simulink model "fdcwind"  (Simulink 3.00)
settings: Solver=ode45  StartTime=0.0  StopTime=50.0  RelTol=1e-3
libraries: airlib x1, simulink3 x1
settings Model: ExtModeTrigMode=normal  ExtModeArmWhenConnect=on  LastModifiedBy=gcampa

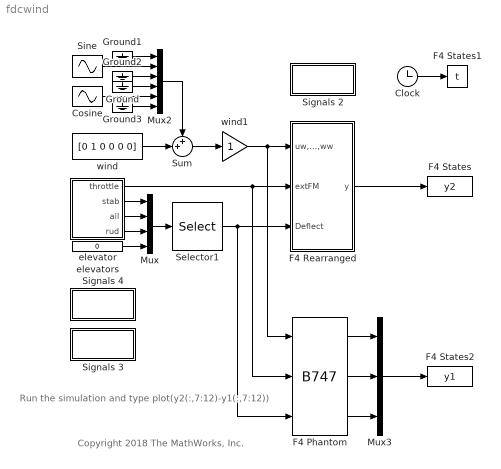
== system fdcwind ==
  note: Run the simulation and type
      | plot(y2(:,7:12)-y1(:,7:12))
  note: Copyright 2018 The MathWorks, Inc.
  " F4 Phantom " : airlib/B747  GM1="[4.8768   11.79576   49.23861   33895.4489   165680.954   189543.35   0   2982.7995  0   17690.1]"  CD_wind="[0.0205  0.3   0  0  -0.1]"  CL_wind="[0.1    3.75    1.8    0    0.4]"  Cm_body="[0.025  -0.4   -2.7    0    -0.58]"  CY_body="[0   -0.68   0     0     0.0160    0.095]"  Cl_body="[0    -0.16    -0.34   0.13    -0.013    0.008]"  Cn_body="[0    0.125   -0.036    -0.270     0.001   -0.066]"  x0="[204.7539671696894 0.0395294 -0.00488392967079  0 0 0   0 0.0395294 0   -70 -20 6065.68]"
  Clock : Clock
      settings: DisplayTime=off  Decimation=10
  Cosine : Sin  Amplitude=1  Frequency=1  Phase=pi/2  SampleTime=0
  F4 Rearranged : Subsystem  mask{GM1=[4.8768   11.79576   49.23861   33895.4489   165680.954   189543.35   0   2982.7995  0   17690.1], CD_wind=[0.0205  0.3   0  0  -0.1], CL_wind=[0.1    3.75    1.8    0    0.4], Cm_body=[0.025  -0.4   -2.7    0    -0.58], CY_body=[0   -0.68   0     0     0.0160    0.095], Cl_body=[0    -0.16    -0.34   0.13    -0.013    0.008], Cn_body=[0    0.125   -0.036    -0.270     0.001   -0.066], x0=[204.7515252  0.0395294 0   0 0 0   0 0.0395294 0   -70 -20 6065.68]}
      mask prompts: GM1 "Geometry and Mass : [cbar   b    S    Ix   Iy   Iz   Jxy  Jxz  Jyz  m]"; CD_wind "Aerodynamic D-Force Coefficients : [CD0 CDa CDq CDde CDih]"; CL_wind "Aerodynamic L-Force Coefficients : [CL0 CLa CLq CLde CLih]"; Cm_body "Aerodynamic Y-Moment Coefficients : [Cm0 Cma Cmq Cmde Cmih]"; CY_body "Aerodynamic Y-Force Coefficients : [CY0 CYb CYp CYr CYda CYdr]"; Cl_body "Aerodynamic X-moment Coefficients : [Cl0 Clb Clp Clr Clda Cldr]"; Cn_body "Aerodynamic Z-moment Coefficients : [Cn0 Cnb Cnp Cnr Cnda Cndr]"; x0 "Initial Condition x0 [v alpha beta p q r psi theta phi xe ye H]"
      mask help:
      | The first input contains the wind velocity and acceleration.
      |   The second input contains external forces and moments in body axis.
      |   The third input contains the deflections of elevators, ailerons, rudder
      |   and, flaps. For a list of outputs look under the mask.
      |   NB : The International measurement system (MKS) is adopted.
      mask init:
      | AM=zeros(6,19);
      | AM(1,[1 2 9 11 12])=reshape(CD_wind,1,5);
      | AM(3,[1 2 9 11 12])=reshape(CL_wind,1,5);
      | AM(5,[1 2 9 11 12])=reshape(Cm_body,1,5);
      | AM(2,[1 5 8 10 13 14])=reshape(CY_body,1,6);
      | AM(4,[1 5 8 10 13 14])=reshape(Cl_body,1,6);
      | AM(6,[1 5 8 10 13 14])=reshape(Cn_body,1,6);
      | 
      | Ix=GM1(4);Iy=GM1(5);Iz=GM1(6);
      | Jxy=GM1(7);Jxz=GM1(8);Jyz=GM1(9);
      | 
      | detI = Ix*Iy*Iz - 2*Jxy*Jxz*Jyz - Ix*Jyz^2 - Iy*Jxz^2 - Iz*Jxy^2;
      | I1   = Iy*Iz - Jyz^2;I2   = Jxy*Iz + Jyz*Jxz;
      | I3   = Jxy*Jyz + Iy*Jxz;I4   = Ix*Iz - Jxz^2;
      | I5   = Ix*Jyz + Jxy*Jxz;I6   = Ix*Iy - Jxy^2;
      | 
      | Pl  = I1/detI; Pm = I2/detI; Pn = I3/detI;
      | Ppp = -(Jxz*I2 - Jxy*I3)/detI;Ppq = (Jxz*I1 - Jyz*I2 - (Iy-Ix)*I3)/detI;
      | Ppr = -(Jxy*I1 + (Ix-Iz)*I2 - Jyz*I3)/detI;Pqq = (Jyz*I1 - Jxy*I3)/detI;
      | Pqr = -((Iz-Iy)*I1 - Jxy*I2 + Jxz*I3)/detI;Prr = -(Jyz*I1 - Jxz*I2)/detI;
      | 
      | Ql  = I2/detI; Qm = I4/detI; Qn = I5/detI;
      | Qpp = -(Jxz*I4 - Jxy*I5)/detI;Qpq = (Jxz*I2 - Jyz*I4 - (Iy-Ix)*I5)/detI;
      | Qpr = -(Jxy*I2 + (Ix-Iz)*I4 - Jyz*I5)/detI;Qqq = (Jyz*I2 - Jxy*I5)/detI;
      | Qqr = -((Iz-Iy)*I2 - Jxy*I4 + Jxz*I5)/detI;Qrr = -(Jyz*I2 - Jxz*I4)/detI;
      | 
      | Rl  = I3/detI; Rm = I5/detI; Rn = I6/detI;
      | Rpp = -(Jxz*I5 - Jxy*I6)/detI;
      | Rpq = (Jxz*I3 - Jyz*I5 - (Iy-Ix)*I6)/detI;
      | Rpr = -(Jxy*I3 + (Ix-Iz)*I5 - Jyz*I6)/detI;
      | Rqq = (Jyz*I3 - Jxy*I6)/detI;
      | Rqr = -((Iz-Iy)*I3 - Jxy*I5 + Jxz*I6)/detI;
      | Rrr = -(Jyz*I3 - Jxz*I5)/detI;
      | 
      | GM2 = [  Pl   Pm   Pn   Ppp  Ppq  Ppr  Pqq  Pqr  Prr ;
      |                Ql  Qm   Qn   Qpp  Qpq  Qpr  Qqq  Qqr  Qrr ;
      |                Rl  Rm   Rn   Rpp  Rpq  Rpr  Rqq  Rqr  Rrr ];
      | 
      | xfix=1;
  F4 States : ToWorkspace  VariableName=y2  SampleTime=0.05  SaveFormat=Matrix
      settings: Buffer=1000
  F4 States1 : ToWorkspace  VariableName=t  SampleTime=0.05  SaveFormat=Matrix
      settings: Buffer=1000
  F4 States2 : ToWorkspace  VariableName=y1  SampleTime=0.05  SaveFormat=Matrix
      settings: Buffer=1000
  Ground{,1..3} (4 alike) : Ground
  Mux : Mux  Inputs=4
      settings: DisplayOption=none
  Mux2 : Mux  Inputs=[1,1,1,1,1,1]
      settings: DisplayOption=none
  Mux3 : Mux  Inputs=3
      settings: DisplayOption=none
  Selector1 : Selector  Elements=[4 2 3 1]  InputPortWidth=4
  Signals 2 : Subsystem
      mask Display: disp('Model \nSignals')
  Signals 3 : Subsystem
      mask Display: disp('Initial \nConditions')
  Signals 4 : Subsystem
      mask Display: disp('INFO')
  Sine : Sin  Amplitude=1  Frequency=1  Phase=0  SampleTime=0
  Sum : Sum  Inputs=++|  SaturateOnIntegerOverflow=on
  elevator : Subsystem
      mask Display: disp('Cable &\nactuator\ndynamics')
  elevators : Constant  Value=0
  wind : Constant  Value=[0 1 0 0 0 0]
  wind1 : Gain  Gain=1  SaturateOnIntegerOverflow=on
  wires:
  elevator/3(ail) -> Mux/2
  elevator/4(rud) -> Mux/3
  elevator/2(stab) -> Mux/1
  Mux/1 -> Selector1/1
  elevators/1 -> Mux/4
  elevator/1(throttle) -> F4 Rearranged/2(extFM), " F4 Phantom "/2
  Selector1/1 -> F4 Rearranged/3(Deflect), " F4 Phantom "/3
  Mux3/1 -> F4 States2/1
  F4 Rearranged/1(y) -> F4 States/1
  wind/1 -> Sum/2
  Clock/1 -> F4 States1/1
  Sine/1 -> Mux2/2
  Ground1/1 -> Mux2/1
  Ground2/1 -> Mux2/3
  Ground/1 -> Mux2/4
  Ground3/1 -> Mux2/6
  Cosine/1 -> Mux2/5
  Mux2/1 -> Sum/1
  Sum/1 -> wind1/1
  wind1/1 -> F4 Rearranged/1(uw,vw,ww), " F4 Phantom "/1
  " F4 Phantom "/1 -> Mux3/1
  " F4 Phantom "/2 -> Mux3/2
  " F4 Phantom "/3 -> Mux3/3

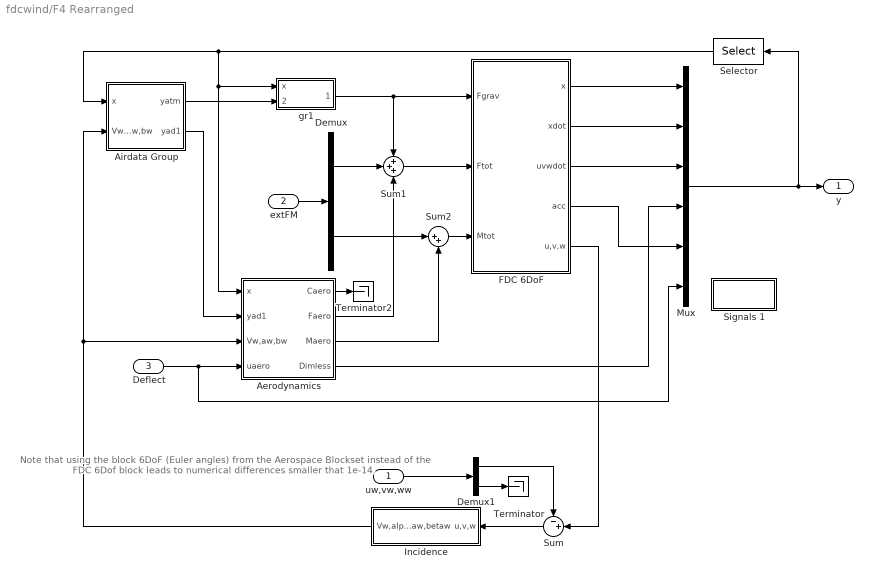
== system fdcwind/F4 Rearranged ==
  note: Note that using the block 6DoF (Euler angles)
      | from the Aerospace Blockset instead of the
      | FDC 6Dof block leads to numerical differences
      | smaller that 1e-14.
  uw,vw,ww : Inport  Port=1  PortWidth=6  SampleTime=-1  DataType=auto
      settings: SignalType=auto
  extFM : Inport  Port=2  PortWidth=6  SampleTime=-1  DataType=auto
      settings: SignalType=auto
  Deflect : Inport  Port=3  PortWidth=-1  SampleTime=-1  DataType=auto
      settings: SignalType=auto
  Aerodynamics : Subsystem
  Airdata Group : Subsystem
  Demux : Demux  Outputs=[3,3]
  Demux1 : Demux  Outputs=[3,3]
  FDC 6DoF : Subsystem
  Incidence : Subsystem  Orientation=left
  Mux : Mux  Inputs=6
  Selector : Selector  Orientation=left  Elements=[1:12]  InputPortWidth=40
  Signals 1 : Subsystem
      mask Display: disp('Output\nSignals')
  Sum : Sum  Orientation=left  Inputs=-+|  SaturateOnIntegerOverflow=on
  Sum1 : Sum  Inputs=+++  SaturateOnIntegerOverflow=on
  Sum2 : Sum  Inputs=|++  SaturateOnIntegerOverflow=on
  Terminator : Terminator
  Terminator2 : Terminator
  gr1 : Subsystem  mask(Gravity){m=GM1(10)}
      mask prompts: m "Mass of the aircraft [kg]:"
      mask help: Gravity forces.
      mask Help: eval('fdchelp gravity')
      mask Display: disp('Gravity')
  y : Outport  Port=1
  wires:
  Aerodynamics/4(Dimless) -> Mux/4
  FDC 6DoF/4(acc) -> Mux/5
  FDC 6DoF/3(uvwdot) -> Mux/3
  FDC 6DoF/2(xdot) -> Mux/2
  FDC 6DoF/1(x) -> Mux/1
  Sum1/1 -> FDC 6DoF/2(Ftot)
  Demux1/2 -> Terminator/1
  Demux1/1 -> Sum/1
  uw,vw,ww/1 -> Demux1/1
  Selector/1 -> Airdata Group/1(x), gr1/1(x), Aerodynamics/1(x)
  Mux/1 -> Selector/1, y/1
  Sum2/1 -> FDC 6DoF/3(Mtot)
  Demux/2 -> Sum2/1
  Aerodynamics/1(Caero) -> Terminator2/1
  Deflect/1 -> Mux/6, Aerodynamics/4(uaero)
  Airdata Group/2(yad1) -> Aerodynamics/2(yad1)
  Incidence/1(Vw,alphaw,betaw) -> Aerodynamics/3(Vw,aw,bw), Airdata Group/2(Vw,aw,bw)
  Sum/1 -> Incidence/1(u,v,w)
  Airdata Group/1(yatm) -> gr1/2(yatm)
  gr1/1(Fgrav) -> FDC 6DoF/1(Fgrav), Sum1/1
  FDC 6DoF/5(u,v,w) -> Sum/2
  extFM/1 -> Demux/1
  Demux/1 -> Sum1/2
  Aerodynamics/2(Faero) -> Sum1/3
  Aerodynamics/3(Maero) -> Sum2/2

== system fdcwind/Signals 2 ==
  note: 01 v (m/s)
      | 02 alpha (rad)
      | 03 beta (rad)
      | 04 p (rad/s)
      | 05 q (rad/s)
      | 06 r  (rad/s)
      | 07 psi (rad)
      | 08 theta (rad)
      | 09 phi (rad)
      | 10 xe (m)
      | 11 ye (m)
      | 12 H (m)
      | 13 v dot (m/s2)
      | 14 alpha dot (rad/s)
      | 15 beta dot (rad/s)
      | 16 p dot (rad/s2)
      | 17 q dot (rad/s2)
      | 18 r dot (rad/s2)
      | 19 psi dot (rad/s)
      | 20 theta dot (rad/s)
      | 21 phi dot (rad/s)
      | 22 xe dot (m/s)
      | 23 ye dot (m/s)
      | 24 H dot (m/s)
      | 25 u dot (m/s2)
      | 26 v dot (m/s2)
      | 27 w dot (m/s2)
      | 28 pb/2v (rad)
      | 29 qc/v (rad)
      | 30 rb/v (rad)
      | 31 Ax (g)
      | 32 Ay (g)
      | 33 Az (g)
      | 34 ax (g)
      | 35 ay (g)
      | 36 az (g)
      | 37 delta elevators (rad)
      | 38 delta ailerons (rad)
      | 39 delta rudder (rad)
      | 40 delta flaps (rad)

== system fdcwind/Signals 3 ==
  note: V=204.7515252;a=0.0395294;b=0;
      | u=V*cos(a)*cos(b);v=V*sin(b);w=V*sin(a)*cos(b);
      |
      | uw=0;vw=1;ww=0;
      |
      | Vw=norm([u v w]-[uw vw ww]);
      | aw=atan((w-ww)/(u-uw));
      | bw=atan((v-vw)/norm([u w]-[uw ww]));
  note: INITIAL CONDITION COMPUTATION FOR
      | THE FDC AIRCRAFT MODEL WITH NONZERO
      | INITIAL WIND

== system fdcwind/Signals 4 ==
  note: This scheme compares two different but
      | equivalent ways to handle the wind
      | inside the equations of motions.
      |
      |
      | It also proves that the way in which FDC handles
      | the wind is fully correct provided that the right
      | initial conditions are chosen for V,alpha,beta
      | whenever the initial value of the wind is nonzero.

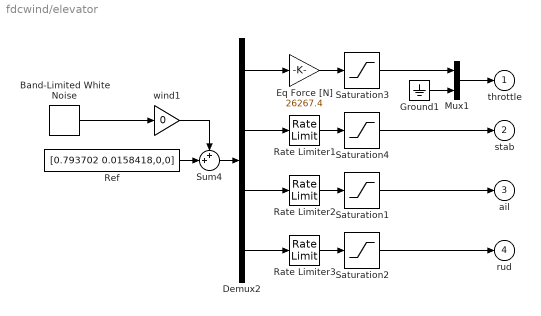
== system fdcwind/elevator ==
  Band-Limited White Noise : simulink3/Sources/Band-Limited White Noise  Cov=0.1*ones(1,4)  Ts=0.1  seed=[1 2 3 4]
  Demux2 : Demux  Outputs=4
  Eq Force [N] : Gain  Gain=26267.4  SaturateOnIntegerOverflow=on
  Ground1 : Ground
  Mux1 : Mux  Inputs=[1 5]
      settings: DisplayOption=none
  Rate Limiter1 : RateLimiter  RisingSlewLimit=100*pi/180  FallingSlewLimit=-100*pi/180
  Rate Limiter2 : RateLimiter  RisingSlewLimit=100*pi/180  FallingSlewLimit=-100*pi/180
  Rate Limiter3 : RateLimiter  RisingSlewLimit=100*pi/180  FallingSlewLimit=-100*pi/180
  Ref : Constant  Value=[0.793702 0.0158418,0,0]
  Saturation1 : Saturate  UpperLimit=20*pi/180  LowerLimit=-20*pi/180
  Saturation2 : Saturate  UpperLimit=20*pi/180  LowerLimit=-20*pi/180
  Saturation3 : Saturate  UpperLimit=52534.8  LowerLimit=0
  Saturation4 : Saturate  UpperLimit=20*pi/180  LowerLimit=-20*pi/180
  Sum4 : Sum  Inputs=++|  SaturateOnIntegerOverflow=on
  wind1 : Gain  Gain=0  SaturateOnIntegerOverflow=on
  throttle : Outport  Port=1
  stab : Outport  Port=2
  ail : Outport  Port=3
  rud : Outport  Port=4
  wires:
  Eq Force [N]/1 -> Saturation3/1
  Ground1/1 -> Mux1/2
  Mux1/1 -> throttle/1
  Saturation3/1 -> Mux1/1
  Ref/1 -> Sum4/2
  Sum4/1 -> Demux2/1
  Rate Limiter1/1 -> Saturation4/1
  Saturation4/1 -> stab/1
  Rate Limiter2/1 -> Saturation1/1
  Saturation1/1 -> ail/1
  Rate Limiter3/1 -> Saturation2/1
  Saturation2/1 -> rud/1
  Demux2/4 -> Rate Limiter3/1
  Demux2/3 -> Rate Limiter2/1
  Demux2/2 -> Rate Limiter1/1
  Demux2/1 -> Eq Force [N]/1
  Band-Limited White Noise/1 -> wind1/1
  wind1/1 -> Sum4/1

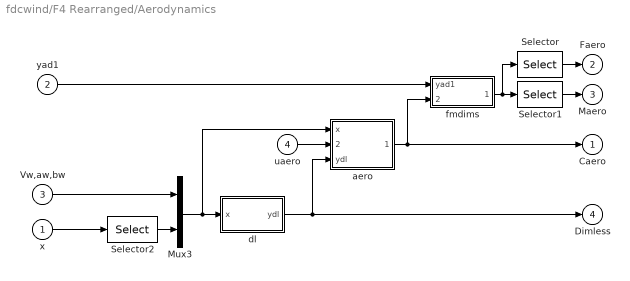
== system fdcwind/F4 Rearranged/Aerodynamics ==
  x : Inport  Port=1  PortWidth=-1  SampleTime=-1  DataType=auto
      settings: SignalType=auto
  yad1 : Inport  Port=2  PortWidth=-1  SampleTime=-1  DataType=auto
      settings: SignalType=auto
  Vw,aw,bw : Inport  Port=3  PortWidth=3  SampleTime=-1  DataType=auto
      settings: SignalType=auto
  uaero : Inport  Port=4  PortWidth=-1  SampleTime=-1  DataType=auto
      settings: SignalType=auto
  Mux3 : Mux  Inputs=2
  Selector : Selector  Elements=[1:3]  InputPortWidth=6
  Selector1 : Selector  Elements=[4:6]  InputPortWidth=6
  Selector2 : Selector  Elements=[4:12]  InputPortWidth=12
  aero : Subsystem
      mask Type: Aeromod
      mask Description: Aerodynamic model of the DHC-2 'Beaver'.
      mask Help: eval('fdchelp aeromod')
      mask Display: disp('Aeromod\n(General)')
  dl : Subsystem  mask(Dimless){cbar=GM1(1), b=GM1(2)}
      mask prompts: cbar "Mean aerodynamic chord [m]:"; b "Wing span [m]:"
      mask help: Dimensionless rotational velocities.
      mask Help: eval('fdchelp dimless')
      mask Display: disp('Dimless')
  fmdims : Subsystem  mask(FMdims){cbar=GM1(1), b=GM1(2), S=GM1(3)}
      mask prompts: cbar "Mean aerodynamic chord [m]:"; b "Wing span [m]:"; S "Wing surface [m^2]:"
      mask help:
      | Calculate forces and moments from
      | dimensionless coefficients.
      mask Help: eval('fdchelp fmdims')
      mask Display: disp('FMdims')
  Caero : Outport  Port=1
  Faero : Outport  Port=2
  Maero : Outport  Port=3
  Dimless : Outport  Port=4
  wires:
  Selector2/1 -> Mux3/2
  Vw,aw,bw/1 -> Mux3/1
  x/1 -> Selector2/1
  Mux3/1 -> aero/1(x), dl/1(x)
  dl/1(ydl) -> Dimless/1, aero/3(ydl)
  aero/1(Caero) -> fmdims/2(Force / moment coefficients), Caero/1
  uaero/1 -> aero/2(uaero)
  yad1/1 -> fmdims/1(yad1)
  fmdims/1(Forces and moments) -> Selector1/1, Selector/1
  Selector1/1 -> Maero/1
  Selector/1 -> Faero/1

== system fdcwind/F4 Rearranged/Airdata Group ==
  x : Inport  Port=1  PortWidth=12  SampleTime=-1  DataType=auto
      settings: SignalType=auto
  Vw,aw,bw : Inport  Port=2  PortWidth=3  SampleTime=-1  DataType=auto
      settings: SignalType=auto
  ad1 : Subsystem
      mask Type: Airdata1
      mask Description: Basic airdata variables
      mask Help: eval('fdchelp airdata1')
      mask Display: disp('Airdata1')
  atm1 : Subsystem
      mask Type: Atmosph
      mask Description:
      | 1-Atmosphere variables
      | 2-Air density
      | 3-Air Pressure
      | 4-Temperature
      | 5-Air viscosity
      | 6-Gravity
      mask Help: eval('fdchelp atmosph')
      mask Display: disp('Atmosph')
  yatm : Outport  Port=1
  yad1 : Outport  Port=2
  wires:
  Vw,aw,bw/1 -> ad1/1(Vw,alphaw,betaw)
  ad1/1(yad1) -> yad1/1
  atm1/1(yatm) -> yatm/1, ad1/2(yatm)
  x/1 -> atm1/1(x)

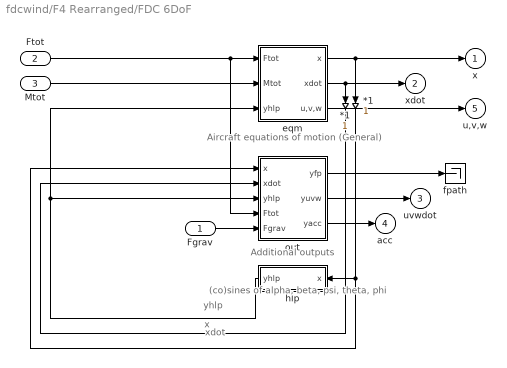
== system fdcwind/F4 Rearranged/FDC 6DoF ==
  note: (co)sines of
      | alpha, beta,
      | psi, theta, phi
  note: Aircraft equations
      | of motion (General)
  note: Additional outputs
  note: yhlp
  note: x
  note: xdot
  Fgrav : Inport  Port=1  PortWidth=3  SampleTime=-1  DataType=auto
      settings: SignalType=auto
  Ftot : Inport  Port=2  PortWidth=3  SampleTime=-1  DataType=auto
      settings: SignalType=auto
  Mtot : Inport  Port=3  PortWidth=3  SampleTime=-1  DataType=auto
      settings: SignalType=auto
  " *1" : Gain  Orientation=down  Gain=1  SaturateOnIntegerOverflow=on
  *1 : Gain  Orientation=down  Gain=1  SaturateOnIntegerOverflow=on
  eqm : Subsystem
  fpath : Terminator
  hlp : Subsystem  Orientation=left
      mask Type: Hlpfcn
      mask Description: Help sines and cosines
      mask Help: eval('fdchelp hlpfcn')
      mask Display: disp('hlpfcn')
  out : Subsystem
  x : Outport  Port=1
  xdot : Outport  Port=2
  uvwdot : Outport  Port=3
  acc : Outport  Port=4
  u,v,w : Outport  Port=5
  wires:
  eqm/3(u,v,w) -> u,v,w/1
  Fgrav/1 -> out/5(Fgrav)
  eqm/2(xdot) -> *1/1, xdot/1
  Mtot/1 -> eqm/2(Mtot)
  Ftot/1 -> eqm/1(Ftot), out/4(Ftot)
  eqm/1(x) -> " *1"/1, x/1
  " *1"/1 -> out/1(x), hlp/1(x)
  out/3(yacc) -> acc/1
  out/1(yfp) -> fpath/1
  out/2(yuvw) -> uvwdot/1
  *1/1 -> out/2(xdot)
  hlp/1(yhlp) -> out/3(yhlp), eqm/3(yhlp)

== system fdcwind/F4 Rearranged/Incidence ==
  u,v,w : Inport  Port=1  PortWidth=3  SampleTime=-1  DataType=auto
      settings: SignalType=auto
  Mux2 : Mux  Inputs=3
  Vrel : Fcn  Expr=sqrt(u[1]^2+u[2]^2+u[3]^2)
  alpha app : Fcn  Expr=atan2(u[3],u[1])
  beta app : Fcn  Expr=atan2(u[2],sqrt(u[1]^2+u[3]^2))
  Vw,alphaw,betaw : Outport  Port=1
  wires:
  Mux2/1 -> Vw,alphaw,betaw/1
  u,v,w/1 -> Vrel/1, alpha app/1, beta app/1
  beta app/1 -> Mux2/3
  alpha app/1 -> Mux2/2
  Vrel/1 -> Mux2/1

== system fdcwind/F4 Rearranged/Signals 1 ==
  note: 01 v (m/s)                        1
      | 02 alpha (rad)                 2
      | 03 beta (rad)                   3
      | 04 p (rad/s)                      4
      | 05 q (rad/s)                      5
      | 06 r  (rad/s)                      6
      | 07 psi (rad)                      7
      | 08 theta (rad)                  8
      | 09 phi (rad)                     9
      | 10 xe (m)
      | 11 ye (m)
      | 12 ze (m)
      | 13 v dot (m/s2)
      | 14 alpha dot (rad/s)
      | 15 beta dot (rad/s)
      | 16 p dot (rad/s2)
      | 17 q dot (rad/s2)
      | 18 r dot (rad/s2)
      | 19 fi dot (rad/s)
      | 20 theta dot (rad/s)
      | 21 psi dot (rad/s)
      | 22 xe dot (m/s)
      | 23 ye dot (m/s)
      | 24 ze dot (m/s)
      | 25 u dot (m/s2)               10
      | 26 v dot (m/s2)               11
      | 27 w dot (m/s2)              12
      | 28 pb/2v (rad)
      | 29 qc/v (rad)
      | 30 rb/v (rad)
      | 31 Ax (g)                        13
      | 32 Ay (g)                        14
      | 33 Az (g)                        15
      | 34 ax (g)                        16
      | 35 ay (g)                        17
      | 36 az (g)                        18
      | 37 delta elevators (rad)  19
      | 38 delta ailerons (rad)    20
      | 39 delta rudder (rad)      21
      | 40 delta flaps (rad)

== system fdcwind/F4 Rearranged/gr1 ==
  x : Inport  Port=1  PortWidth=-1  SampleTime=-1  DataType=auto
      settings: SignalType=auto
  yatm : Inport  Port=2  PortWidth=-1  SampleTime=-1  DataType=auto
      settings: SignalType=auto
  0 : Subsystem
      settings: OpenFcn=fdchelp gravity
      mask Display: disp('GRAVITY\nM.O. Rauw, October 1997')
  Mux : Mux  Inputs=3
      settings: DisplayOption=none
  Mux1 : Mux  Inputs=[12 5]
      settings: DisplayOption=none
  Xgr : Fcn  Expr=-m*u[17]*sin(u[8])
  Ygr : Fcn  Expr=m*u[17]*cos(u[8])*sin(u[9])
  Zgr : Fcn  Expr=m*u[17]*cos(u[8])*cos(u[9])
  Fgrav : Outport  Port=1
  wires:
  yatm/1 -> Mux1/2
  x/1 -> Mux1/1
  Zgr/1 -> Mux/3
  Mux1/1 -> Zgr/1, Xgr/1, Ygr/1
  Mux/1 -> Fgrav/1
  Ygr/1 -> Mux/2
  Xgr/1 -> Mux/1

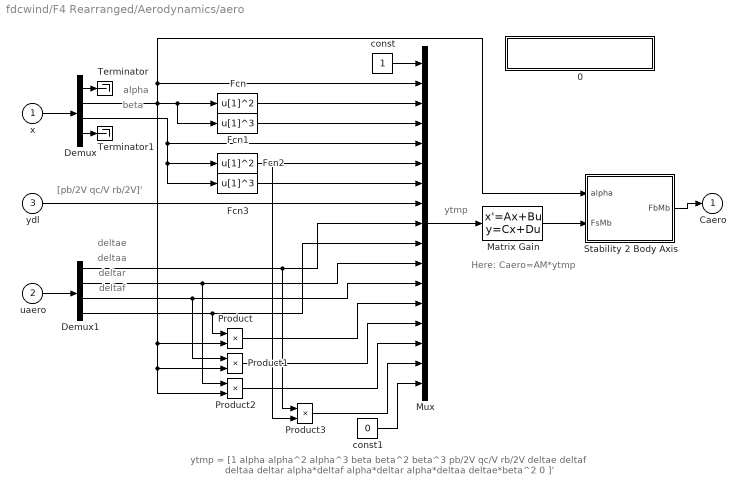
== system fdcwind/F4 Rearranged/Aerodynamics/aero ==
  note: Here: Caero=AM*ytmp
  note: ytmp
  note: alpha
  note: deltaf
  note: deltar
  note: deltaa
  note: deltae
  note: beta
  note: [pb/2V qc/V rb/2V]'
  note: ytmp = [1  alpha  alpha^2  alpha^3  beta  beta^2  beta^3  pb/2V  qc/V  rb/2V  deltae
      | deltaf  deltaa  deltar  alpha*deltaf  alpha*deltar  alpha*deltaa  deltae*beta^2  0 ]'
  x : Inport  Port=1  PortWidth=-1  SampleTime=-1  DataType=auto
      settings: SignalType=auto
  uaero : Inport  Port=2  PortWidth=-1  SampleTime=-1  DataType=auto
      settings: SignalType=auto
  ydl : Inport  Port=3  PortWidth=-1  SampleTime=-1  DataType=auto
      settings: SignalType=auto
  0 : Subsystem
      settings: OpenFcn=fdchelp aeromod
      mask Display: disp('AEROMOD\nM.O. Rauw, October 1997')
  Demux : Demux  Outputs=[1 1 1 9]
  Demux1 : Demux  Outputs=4
  Fcn : Fcn  Expr=u[1]^2
  Fcn1 : Fcn  Expr=u[1]^3
  Fcn2 : Fcn  Expr=u[1]^2
  Fcn3 : Fcn  Expr=u[1]^3
  Matrix Gain : StateSpace  A=[]  B=[]  C=[]  D=AM  X0=0
  Mux : Mux  Inputs=[1 1 1 1 1 1 1 3 1 1 1 1 1 1 1 1 1]
      settings: DisplayOption=none
  Product{,1..3} (4 alike) : Product  Inputs=2  SaturateOnIntegerOverflow=on
  Stability 2 Body Axis : Subsystem
  Terminator : Terminator
  Terminator1 : Terminator
  const : Constant  Value=1
  const1 : Constant  Value=0
  Caero : Outport  Port=1
  wires:
  Matrix Gain/1 -> Stability 2 Body Axis/2(FsMb)
  Stability 2 Body Axis/1(FbMb) -> Caero/1
  Mux/1 -> Matrix Gain/1
  x/1 -> Demux/1
  Fcn/1 -> Mux/3
  Fcn1/1 -> Mux/4
  uaero/1 -> Demux1/1
  Fcn3/1 -> Mux/7
  Product/1 -> Mux/13
  Demux1/3 -> Product1/1, Mux/12
  Demux1/2 -> Product2/1, Mux/11
  Demux/3 -> Fcn3/1, Fcn2/1, Mux/5
  Demux/2 -> Stability 2 Body Axis/1(alpha), Mux/2, Product2/2, Product1/2, Product/2, Fcn1/1, Fcn/1
  Demux1/4 -> Product/1, Mux/10
  Fcn2/1 -> Product3/2, Mux/6
  Demux1/1 -> Product3/1, Mux/9
  Product1/1 -> Mux/14
  Product2/1 -> Mux/15
  Product3/1 -> Mux/16
  ydl/1 -> Mux/8
  const/1 -> Mux/1
  const1/1 -> Mux/17
  Demux/1 -> Terminator/1
  Demux/4 -> Terminator1/1

== system fdcwind/F4 Rearranged/Aerodynamics/dl ==
  x : Inport  Port=1  PortWidth=-1  SampleTime=-1  DataType=auto
      settings: SignalType=auto
  0 : Subsystem
      settings: OpenFcn=fdchelp dimless
      mask Display: disp('DIMLESS\nM.O. Rauw, October 1997')
  Mux : Mux  Inputs=3
      settings: DisplayOption=none
  pb/2V : Fcn  Expr=0.5 * u[4] * b / u[1]
  qc/2V : Fcn  Expr=0.5* u[5] * cbar / u[1]
  rb/2V : Fcn  Expr=0.5 * u[6] * b / u[1]
  ydl : Outport  Port=1
  wires:
  x/1 -> pb/2V/1, rb/2V/1, qc/2V/1
  Mux/1 -> ydl/1
  rb/2V/1 -> Mux/3
  qc/2V/1 -> Mux/2
  pb/2V/1 -> Mux/1

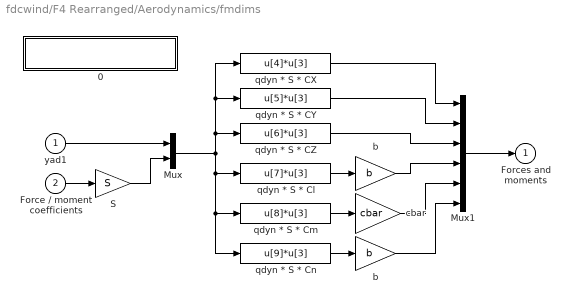
== system fdcwind/F4 Rearranged/Aerodynamics/fmdims ==
  yad1 : Inport  Port=1  PortWidth=-1  SampleTime=-1  DataType=auto
      settings: SignalType=auto
  Force / moment coefficients : Inport  Port=2  PortWidth=-1  SampleTime=-1  DataType=auto
      settings: SignalType=auto
  0 : Subsystem
      settings: OpenFcn=fdchelp fmdims
      mask Display: disp('FMDIMS\nM.O. Rauw, October 1997')
  Mux : Mux  Inputs=[3 6]
      settings: DisplayOption=none
  Mux1 : Mux  Inputs=6
      settings: DisplayOption=none
  S : Gain  Gain=S  SaturateOnIntegerOverflow=on
  b : Gain  Gain=b  SaturateOnIntegerOverflow=on
  "b " : Gain  Gain=b  SaturateOnIntegerOverflow=on
  cbar : Gain  Gain=cbar  SaturateOnIntegerOverflow=on
  qdyn * S * CX : Fcn  Expr=u[4]*u[3]
  qdyn * S * CY : Fcn  Expr=u[5]*u[3]
  qdyn * S * CZ : Fcn  Expr=u[6]*u[3]
  qdyn * S * Cl : Fcn  Expr=u[7]*u[3]
  qdyn * S * Cm : Fcn  Expr=u[8]*u[3]
  qdyn * S * Cn : Fcn  Expr=u[9]*u[3]
  Forces and moments : Outport  Port=1
  wires:
  b/1 -> Mux1/4
  qdyn * S * CZ/1 -> Mux1/3
  S/1 -> Mux/2
  qdyn * S * CY/1 -> Mux1/2
  qdyn * S * CX/1 -> Mux1/1
  yad1/1 -> Mux/1
  qdyn * S * Cn/1 -> "b "/1
  qdyn * S * Cm/1 -> cbar/1
  qdyn * S * Cl/1 -> b/1
  Mux/1 -> qdyn * S * Cn/1, qdyn * S * Cm/1, qdyn * S * Cl/1, qdyn * S * CY/1, qdyn * S * CX/1, qdyn * S * CZ/1
  Force / moment coefficients/1 -> S/1
  cbar/1 -> Mux1/5
  "b "/1 -> Mux1/6
  Mux1/1 -> Forces and moments/1

== system fdcwind/F4 Rearranged/Airdata Group/ad1 ==
  Vw,alphaw,betaw : Inport  Port=1  PortWidth=-1  SampleTime=-1  DataType=auto
      settings: SignalType=auto
  yatm : Inport  Port=2  PortWidth=-1  SampleTime=-1  DataType=auto
      settings: SignalType=auto
  0 : Subsystem
      settings: OpenFcn=fdchelp airdata1
      mask Display: disp('AIRDATA1\nM.O. Rauw, October 1997')
  M : Fcn  Expr=u[2]/u[1]
  Mux : Mux  Inputs=[1 3]
      settings: DisplayOption=none
  Mux1 : Mux  Inputs=[3 5]
      settings: DisplayOption=none
  Mux2 : Mux  Inputs=3
      settings: DisplayOption=none
  a : Fcn  Expr=sqrt(401.8743*u[3])
  qdyn : Fcn  Expr=0.5*u[4]*u[1]^2
  yad1 : Outport  Port=1
  wires:
  yatm/1 -> Mux1/2, a/1
  Vw,alphaw,betaw/1 -> Mux1/1, Mux/2
  Mux/1 -> M/1
  Mux1/1 -> qdyn/1
  M/1 -> Mux2/2
  a/1 -> Mux2/1, Mux/1
  qdyn/1 -> Mux2/3
  Mux2/1 -> yad1/1

== system fdcwind/F4 Rearranged/Airdata Group/atm1 ==
  x : Inport  Port=1  PortWidth=-1  SampleTime=-1  DataType=auto
      settings: SignalType=auto
  0 : Subsystem
      settings: OpenFcn=fdchelp atmosph
      mask Display: disp('ATMOSPH\nM.O. Rauw, October 1997')
  Mux : Mux  Inputs=2
      settings: DisplayOption=none
  Mux1 : Mux  Inputs=[2 1]
      settings: DisplayOption=none
  Mux2 : Mux  Inputs=5
      settings: DisplayOption=none
  T : Fcn  Expr=288.15 - 0.0065*u[12]
  g : Fcn  Expr=9.80665*(6371020/(6371020+u[12]))^2
  mu : Fcn  Expr=(1.458*10^(-6)*u[2]^1.5)/(u[2]+110.4)
  ps : Fcn  Expr=101325*(u[2]/288.15)^(u[1]/1.86584)
  rho : Fcn  Expr=u[3]/(287.053*u[2])
  yatm : Outport  Port=1
  wires:
  mu/1 -> Mux2/4
  Mux2/1 -> yatm/1
  Mux1/1 -> rho/1
  rho/1 -> Mux2/1
  g/1 -> Mux2/5, Mux/1
  T/1 -> Mux2/3, Mux/2
  ps/1 -> Mux2/2, Mux1/2
  Mux/1 -> ps/1, mu/1, Mux1/1
  x/1 -> g/1, T/1

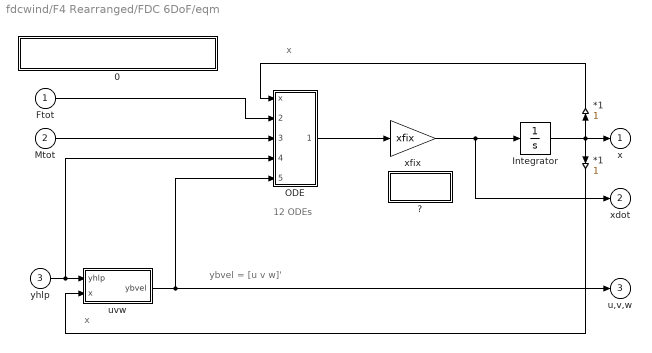
== system fdcwind/F4 Rearranged/FDC 6DoF/eqm ==
  note: 12 ODEs
  note: ybvel = [u v w]'
  note: x
  note: x
  Ftot : Inport  Port=1  PortWidth=-1  SampleTime=-1  DataType=auto
      settings: SignalType=auto
  Mtot : Inport  Port=2  PortWidth=-1  SampleTime=-1  DataType=auto
      settings: SignalType=auto
  yhlp : Inport  Port=3  PortWidth=-1  SampleTime=-1  DataType=auto
      settings: SignalType=auto
  " *1" : Gain  Orientation=up  Gain=1  SaturateOnIntegerOverflow=on
  *1 : Gain  Orientation=down  Gain=1  SaturateOnIntegerOverflow=on
  0 : Subsystem
      settings: OpenFcn=fdchelp eqmotion
      mask Display: disp('EQUATIONS OF MOTION (level 3)\nM.O. Rauw')
  "?" : Subsystem
      settings: OpenFcn=fdchelp xfix
      mask Display: disp('More info\nfor xfix')
  Integrator : Integrator  ExternalReset=none  InitialConditionSource=internal  InitialCondition=x0  LimitOutput=off  UpperSaturationLimit=inf  LowerSaturationLimit=-inf  ShowSaturationPort=off  ShowStatePort=off  AbsoluteTolerance=auto
  ODE : Subsystem
  uvw : Subsystem
      mask Type: uvw
      mask Description:
      | Calculation of body-axes velocities
      | u, v, and w
      mask Help: eval('fdchelp uvw')
      mask Display: disp('Body-axes\nvelocities')
  xfix : Gain  Gain=xfix  SaturateOnIntegerOverflow=on
  x : Outport  Port=1
  xdot : Outport  Port=2
  u,v,w : Outport  Port=3
  wires:
  *1/1 -> uvw/2(x)
  Mtot/1 -> ODE/3(Mtot)
  Ftot/1 -> ODE/2(Ftot)
  uvw/1(ybvel) -> ODE/5(ybvel*), u,v,w/1
  yhlp/1 -> uvw/1(yhlp), ODE/4(yhlp)
  " *1"/1 -> ODE/1(x)
  Integrator/1 -> *1/1, " *1"/1, x/1
  ODE/1(xdot) -> xfix/1
  xfix/1 -> Integrator/1, xdot/1

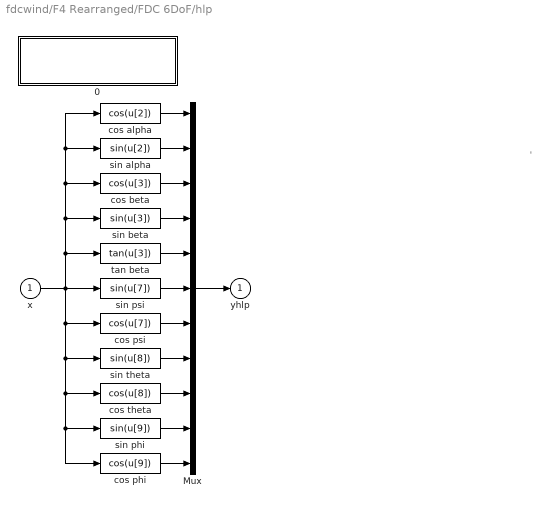
== system fdcwind/F4 Rearranged/FDC 6DoF/hlp ==
  note: '
  x : Inport  Port=1  PortWidth=-1  SampleTime=-1  DataType=auto
      settings: SignalType=auto
  0 : Subsystem
      settings: OpenFcn=fdchelp hlpfcn
      mask Display: disp('HELP FUNCTIONS\n(often used sines and cosines)\nM.O. Rauw, October 1997')
  Mux : Mux  Inputs=11
      settings: DisplayOption=none
  cos alpha : Fcn  Expr=cos(u[2])
  cos beta : Fcn  Expr=cos(u[3])
  cos phi : Fcn  Expr=cos(u[9])
  cos psi : Fcn  Expr=cos(u[7])
  cos theta : Fcn  Expr=cos(u[8])
  sin alpha : Fcn  Expr=sin(u[2])
  sin beta : Fcn  Expr=sin(u[3])
  sin phi : Fcn  Expr=sin(u[9])
  sin psi : Fcn  Expr=sin(u[7])
  sin theta : Fcn  Expr=sin(u[8])
  tan beta : Fcn  Expr=tan(u[3])
  yhlp : Outport  Port=1
  wires:
  cos phi/1 -> Mux/11
  Mux/1 -> yhlp/1
  sin phi/1 -> Mux/10
  cos theta/1 -> Mux/9
  sin theta/1 -> Mux/8
  cos psi/1 -> Mux/7
  sin psi/1 -> Mux/6
  tan beta/1 -> Mux/5
  sin beta/1 -> Mux/4
  cos beta/1 -> Mux/3
  sin alpha/1 -> Mux/2
  cos alpha/1 -> Mux/1
  x/1 -> cos psi/1, cos phi/1, sin phi/1, cos theta/1, sin theta/1, tan beta/1, cos alpha/1, sin alpha/1, cos beta/1, sin beta/1, sin psi/1

== system fdcwind/F4 Rearranged/FDC 6DoF/out ==
  note: Body-axes accelerations
      | and specific forces
  note: du/dt, dv/dt, dw/dt
      | (output equations!)
  note: Flightpath
      | variables
  x : Inport  Port=1  PortWidth=-1  SampleTime=-1  DataType=auto
      settings: SignalType=auto
  xdot : Inport  Port=2  PortWidth=-1  SampleTime=-1  DataType=auto
      settings: SignalType=auto
  yhlp : Inport  Port=3  PortWidth=-1  SampleTime=-1  DataType=auto
      settings: SignalType=auto
  Ftot : Inport  Port=4  PortWidth=-1  SampleTime=-1  DataType=auto
      settings: SignalType=auto
  Fgrav : Inport  Port=5  PortWidth=-1  SampleTime=-1  DataType=auto
      settings: SignalType=auto
  0 : Subsystem
      settings: OpenFcn=fdchelp moreouts
      mask Display: disp('Additional outputs (level 3)\nM.O. Rauw')
  accel : Subsystem  mask(accel){m=GM1(10)}
      mask prompts: m "Mass of the aircraft [kg]:"
      mask help:
      | Body axes accelerations and
      | specific forces.
      mask Help: eval('fdchelp accel')
      mask Display: disp('Accel')
  fp : Subsystem  mask(Flpath){alpha0=x0(2)}
      mask prompts: alpha0 "Initial value of angle of attack, alpha0:"
      mask help: Flightpath related parameters.
      mask Help: eval('fdchelp flpath')
      mask Display: disp('flpath')
  uvwdot : Subsystem
      mask Type: uvwdot
      mask Description: Calculation of du/dt, dv/dt, and dw/dt.
      mask Help: eval('fdchelp uvwdot')
      mask Display: disp('uvwdot')
  yfp : Outport  Port=1
  yuvw : Outport  Port=2
  yacc : Outport  Port=3
  wires:
  Fgrav/1 -> accel/2(Fgrav)
  x/1 -> uvwdot/1(x), fp/1(x)
  xdot/1 -> uvwdot/2(xdot), fp/2(xdot)
  accel/1(yacc) -> yacc/1
  Ftot/1 -> accel/1(Ftot)
  yhlp/1 -> uvwdot/3(yhlp)
  uvwdot/1(yuvw =  [udot; vdot; wdot]) -> yuvw/1
  fp/1(yfp) -> yfp/1

== system fdcwind/F4 Rearranged/gr1/0 ==

== system fdcwind/F4 Rearranged/Aerodynamics/aero/0 ==

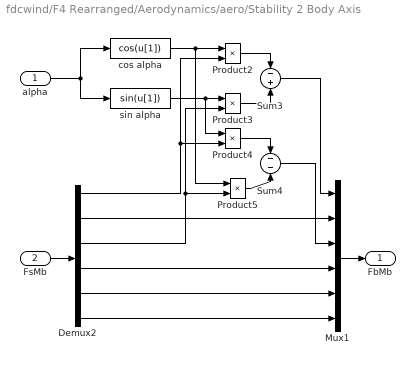
== system fdcwind/F4 Rearranged/Aerodynamics/aero/Stability 2 Body Axis ==
  alpha : Inport  Port=1  PortWidth=-1  SampleTime=-1  DataType=auto
      settings: SignalType=auto
  FsMb : Inport  Port=2  PortWidth=-1  SampleTime=-1  DataType=auto
      settings: SignalType=auto
  Demux2 : Demux  Outputs=6
  Mux1 : Mux  Inputs=6
      settings: DisplayOption=none
  Product{2..5} (4 alike) : Product  Inputs=2  SaturateOnIntegerOverflow=on
  Sum3 : Sum  Inputs=-+  SaturateOnIntegerOverflow=on
  Sum4 : Sum  Inputs=--  SaturateOnIntegerOverflow=on
  cos alpha : Fcn  Expr=cos(u[1])
  sin alpha : Fcn  Expr=sin(u[1])
  FbMb : Outport  Port=1
  wires:
  FsMb/1 -> Demux2/1
  Mux1/1 -> FbMb/1
  alpha/1 -> cos alpha/1, sin alpha/1
  Sum4/1 -> Mux1/3
  Product5/1 -> Sum4/2
  Product4/1 -> Sum4/1
  Demux2/3 -> Product5/2, Product3/2
  sin alpha/1 -> Product4/1, Product3/1
  Sum3/1 -> Mux1/1
  Product3/1 -> Sum3/2
  Product2/1 -> Sum3/1
  Demux2/1 -> Product4/2, Product2/2
  cos alpha/1 -> Product5/1, Product2/1
  Demux2/4 -> Mux1/4
  Demux2/2 -> Mux1/2
  Demux2/5 -> Mux1/5
  Demux2/6 -> Mux1/6

== system fdcwind/F4 Rearranged/Aerodynamics/dl/0 ==

== system fdcwind/F4 Rearranged/Aerodynamics/fmdims/0 ==

== system fdcwind/F4 Rearranged/Airdata Group/ad1/0 ==

== system fdcwind/F4 Rearranged/Airdata Group/atm1/0 ==

== system fdcwind/F4 Rearranged/FDC 6DoF/eqm/0 ==

== system fdcwind/F4 Rearranged/FDC 6DoF/eqm/? ==

== system fdcwind/F4 Rearranged/FDC 6DoF/eqm/ODE ==
  x : Inport  Port=1  PortWidth=-1  SampleTime=-1  DataType=auto
      settings: SignalType=auto
  Ftot : Inport  Port=2  PortWidth=-1  SampleTime=-1  DataType=auto
      settings: SignalType=auto
  Mtot : Inport  Port=3  PortWidth=-1  SampleTime=-1  DataType=auto
      settings: SignalType=auto
  yhlp : Inport  Port=4  PortWidth=-1  SampleTime=-1  DataType=auto
      settings: SignalType=auto
  ybvel* : Inport  Port=5  PortWidth=-1  SampleTime=-1  DataType=auto
      settings: SignalType=auto
  0 : Subsystem
      settings: OpenFcn=fdchelp 12odes
      mask Display: disp('12 Ordinary Differential\nEquations (level 4)\nM.O. Rauw')
  Eulerdot : Subsystem
      mask Type: Eulerdot
      mask Description:
      | Calculation of d(psi)/dt, d(theta)/dt,
      | and d(phi/dt)
      mask Help: eval('fdchelp eulerdot')
      mask Display: disp('psi dot\ntheta dot\nphi dot')
  Mux : Mux  Inputs=[12 3 3 11]
      settings: DisplayOption=none
  Mux1 : Mux  Inputs=[3 3 3 3]
      settings: DisplayOption=none
  Vabdot : Subsystem  mask(Vabdot){m=GM1(10)}
      mask prompts: m "Mass of the aircraft [kg]:"
      mask help: Calculation of dV/dt, dalpha/dt, dbeta/dt.
      mask Help: eval('fdchelp vabdot')
      mask Display: disp('V dot\nalpha dot\nbeta dot')
  pqrdot : Subsystem
      mask Type: pqrdot
      mask Description: Calculation of dp/dt, dq/dt, and dr/dt
      mask Help: eval('fdchelp pqrdot')
      mask Display: disp('p dot\nq dot\nr dot')
  xyHdot : Subsystem
      mask Type: xyHdot
      mask Description: Calculation of d(xe)/dt, d(ye)/dt, and dH/dt
      mask Help: eval('fdchelp xyhdot')
      mask Display: disp('xe dot\nye dot\nH dot')
  xdot : Outport  Port=1
  wires:
  Mux1/1 -> xdot/1
  Vabdot/1(yVab) -> Mux1/1
  pqrdot/1(ypqr) -> Mux1/2
  Eulerdot/1(yeul) -> Mux1/3
  xyHdot/1(yxyH) -> Mux1/4
  yhlp/1 -> Mux/4
  ybvel*/1 -> xyHdot/1(ybvel*)
  Mux/1 -> xyHdot/2(uxYH), Eulerdot/1(ueul), Vabdot/1(uVab), pqrdot/1(upqr)
  Ftot/1 -> Mux/2
  Mtot/1 -> Mux/3
  x/1 -> Mux/1

== system fdcwind/F4 Rearranged/FDC 6DoF/eqm/uvw ==
  yhlp : Inport  Port=1  PortWidth=-1  SampleTime=-1  DataType=auto
      settings: SignalType=auto
  x : Inport  Port=2  PortWidth=-1  SampleTime=-1  DataType=auto
      settings: SignalType=auto
  0 : Subsystem
      settings: OpenFcn=fdchelp uvw
      mask Display: disp('UVW\nM.O. Rauw, October 1997')
  Mux : Mux  Inputs=3
      settings: DisplayOption=none
  Mux1 : Mux  Inputs=[12 11]
      settings: DisplayOption=none
  u : Fcn  Expr=u[1]*u[13]*u[15]
  v : Fcn  Expr=u[1]*u[16]
  w : Fcn  Expr=u[1]*u[14]*u[15]
  ybvel : Outport  Port=1
  wires:
  Mux/1 -> ybvel/1
  w/1 -> Mux/3
  v/1 -> Mux/2
  u/1 -> Mux/1
  x/1 -> Mux1/1
  yhlp/1 -> Mux1/2
  Mux1/1 -> w/1, u/1, v/1

== system fdcwind/F4 Rearranged/FDC 6DoF/hlp/0 ==

== system fdcwind/F4 Rearranged/FDC 6DoF/out/0 ==

== system fdcwind/F4 Rearranged/FDC 6DoF/out/accel ==
  Ftot : Inport  Port=1  PortWidth=-1  SampleTime=-1  DataType=auto
      settings: SignalType=auto
  Fgrav : Inport  Port=2  PortWidth=-1  SampleTime=-1  DataType=auto
      settings: SignalType=auto
  0 : Subsystem
      settings: OpenFcn=fdchelp accel
      mask Display: disp('ACCEL\nM.O. Rauw, October 1997')
  Ax : Fcn  Expr=(u[1]-u[4])/(m*9.80665)
  Ay : Fcn  Expr=(u[2]-u[5])/(m*9.80665)
  Az : Fcn  Expr=(u[3]-u[6])/(m*9.80665)
  Mux : Mux  Inputs=6
      settings: DisplayOption=none
  Mux1 : Mux  Inputs=[3 3]
      settings: DisplayOption=none
  axk : Fcn  Expr=u[1]/(m*9.80665)
  ayk : Fcn  Expr=u[2]/(m*9.80665)
  azk : Fcn  Expr=u[3]/(m*9.80665)
  yacc : Outport  Port=1
  wires:
  ayk/1 -> Mux/5
  axk/1 -> Mux/4
  Mux1/1 -> ayk/1, azk/1, axk/1, Ay/1, Ax/1, Az/1
  Ax/1 -> Mux/1
  Ay/1 -> Mux/2
  Az/1 -> Mux/3
  azk/1 -> Mux/6
  Mux/1 -> yacc/1
  Fgrav/1 -> Mux1/2
  Ftot/1 -> Mux1/1

== system fdcwind/F4 Rearranged/FDC 6DoF/out/fp ==
  x : Inport  Port=1  PortWidth=-1  SampleTime=-1  DataType=auto
      settings: SignalType=auto
  xdot : Inport  Port=2  PortWidth=-1  SampleTime=-1  DataType=auto
      settings: SignalType=auto
  0 : Subsystem
      settings: OpenFcn=fdchelp flpath
      mask Display: disp('FLPATH\nM.O. Rauw, October 1997')
  Mux : Mux  Inputs=[12 12]
      settings: DisplayOption=none
  Mux1 : Mux  Inputs=4
      settings: DisplayOption=none
  Phi : Fcn  Expr=u[9]*cos(u[8]-alpha0)
  chi : Fcn  Expr=u[3]+u[7]
  fpa : Fcn  Expr=u[13]/9.80665
  gamma : Fcn  Expr=asin(u[24]/u[1])
  yfp : Outport  Port=1
  wires:
  xdot/1 -> Mux/2
  x/1 -> Mux/1
  Mux1/1 -> yfp/1
  Phi/1 -> Mux1/4
  chi/1 -> Mux1/3
  fpa/1 -> Mux1/2
  Mux/1 -> gamma/1, fpa/1, Phi/1, chi/1
  gamma/1 -> Mux1/1

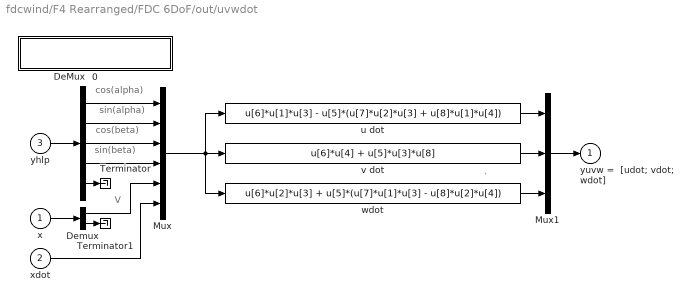
== system fdcwind/F4 Rearranged/FDC 6DoF/out/uvwdot ==
  note: V
  note: sin(beta)
  note: cos(beta)
  note: sin(alpha)
  note: cos(alpha)
  note: `
  x : Inport  Port=1  PortWidth=-1  SampleTime=-1  DataType=auto
      settings: SignalType=auto
  xdot : Inport  Port=2  PortWidth=-1  SampleTime=-1  DataType=auto
      settings: SignalType=auto
  yhlp : Inport  Port=3  PortWidth=-1  SampleTime=-1  DataType=auto
      settings: SignalType=auto
  0 : Subsystem
      settings: OpenFcn=fdchelp uvwdot
      mask Display: disp('UVWDOT\nM.O. Rauw, October 1997')
  DeMux : Demux  Outputs=[1 1 1 1 7]
  Demux : Demux  Outputs=[1 11]
  Mux : Mux  Inputs=[1 1 1 1 1 12]
      settings: DisplayOption=none
  Mux1 : Mux  Inputs=3
      settings: DisplayOption=none
  Terminator : Terminator
  Terminator1 : Terminator
  u dot : Fcn  Expr=u[6]*u[1]*u[3] - u[5]*(u[7]*u[2]*u[3] + u[8]*u[1]*u[4])
  v dot : Fcn  Expr=u[6]*u[4] + u[5]*u[3]*u[8]
  wdot : Fcn  Expr=u[6]*u[2]*u[3] + u[5]*(u[7]*u[1]*u[3] - u[8]*u[2]*u[4])
  yuvw =  [udot; vdot; wdot] : Outport  Port=1
  wires:
  Demux/1 -> Mux/5
  DeMux/4 -> Mux/4
  DeMux/3 -> Mux/3
  yhlp/1 -> DeMux/1
  Mux1/1 -> yuvw =  [udot; vdot; wdot]/1
  x/1 -> Demux/1
  DeMux/2 -> Mux/2
  DeMux/1 -> Mux/1
  Mux/1 -> u dot/1, wdot/1, v dot/1
  xdot/1 -> Mux/6
  u dot/1 -> Mux1/1
  v dot/1 -> Mux1/2
  wdot/1 -> Mux1/3
  DeMux/5 -> Terminator/1
  Demux/2 -> Terminator1/1

== system fdcwind/F4 Rearranged/FDC 6DoF/eqm/ODE/0 ==

== system fdcwind/F4 Rearranged/FDC 6DoF/eqm/ODE/Eulerdot ==
  note: yeul=[psi dot; theta dot; phi dot]
  note: ueul=[x;Ftot;Mtot;yhlp]
  ueul : Inport  Port=1  PortWidth=-1  SampleTime=-1  DataType=auto
      settings: SignalType=auto
  0 : Subsystem
      settings: OpenFcn=fdchelp eulerdot
      mask Display: disp('EULERDOT\nM.O. Rauw, October 1997')
  Mux1 : Mux  Inputs=[29 1]
      settings: DisplayOption=none
  Mux2 : Mux  Inputs=3
      settings: DisplayOption=none
  phi dot : Fcn  Expr=u[4] + u[30]*u[26]
  psi dot : Fcn  Expr=(u[5]*u[28] + u[6]*u[29])/u[27]
  theta dot : Fcn  Expr=u[5]*u[29] - u[6]*u[28]
  yeul : Outport  Port=1
  wires:
  Mux1/1 -> phi dot/1
  phi dot/1 -> Mux2/3
  Mux2/1 -> yeul/1
  theta dot/1 -> Mux2/2
  psi dot/1 -> Mux1/2, Mux2/1
  ueul/1 -> psi dot/1, Mux1/1, theta dot/1

== system fdcwind/F4 Rearranged/FDC 6DoF/eqm/ODE/Vabdot ==
  note: uVab=[x;Ftot;Mtot;yhlp]
  note: yVab=[V dot;alpha dot;beta dot]
  uVab : Inport  Port=1  PortWidth=-1  SampleTime=-1  DataType=auto
      settings: SignalType=auto
  0 : Subsystem
      settings: OpenFcn=fdchelp vabdot
      mask Display: disp('VABDOT\nM.O. Rauw, October 1997')
  Mux2 : Mux  Inputs=3
      settings: DisplayOption=none
  V dot : Fcn  Expr=(u[13]*u[19]*u[21]+u[14]*u[22]+u[15]*u[20]*u[21])/m
  alpha dot : Fcn  Expr=(-u[13]*u[20]+u[15]*u[19])/(m*u[1]*u[21]) - u[23]*(u[4]*u[19]+u[6]*u[20]) + u[5]
  beta dot : Fcn  Expr=(-u[13]*u[19]*u[22]+u[14]*u[21]-u[15]*u[20]*u[22])/(m*u[1]) + u[4]*u[20] - u[6]*u[19]
  yVab : Outport  Port=1
  wires:
  Mux2/1 -> yVab/1
  uVab/1 -> V dot/1, beta dot/1, alpha dot/1
  alpha dot/1 -> Mux2/2
  V dot/1 -> Mux2/1
  beta dot/1 -> Mux2/3

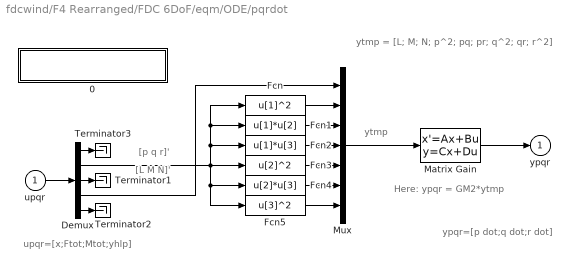
== system fdcwind/F4 Rearranged/FDC 6DoF/eqm/ODE/pqrdot ==
  note: [p q r]'
  note: [L M N]'
  note: Here: ypqr = GM2*ytmp
  note: ytmp
  note: ypqr=[p dot;q dot;r dot]
  note: upqr=[x;Ftot;Mtot;yhlp]
  note: ytmp = [L; M; N; p^2; pq; pr; q^2; qr; r^2]
  upqr : Inport  Port=1  PortWidth=-1  SampleTime=-1  DataType=auto
      settings: SignalType=auto
  0 : Subsystem
      settings: OpenFcn=fdchelp pqrdot
      mask Display: disp('PQRDOT\nM.O. Rauw, October 1997')
  Demux : Demux  Outputs=[3 3 9 3 11]
  Fcn : Fcn  Expr=u[1]^2
  Fcn1 : Fcn  Expr=u[1]*u[2]
  Fcn2 : Fcn  Expr=u[1]*u[3]
  Fcn3 : Fcn  Expr=u[2]^2
  Fcn4 : Fcn  Expr=u[2]*u[3]
  Fcn5 : Fcn  Expr=u[3]^2
  Matrix Gain : StateSpace  A=[]  B=[]  C=[]  D=GM2  X0=0
  Mux : Mux  Inputs=[3 1 1 1 1 1 1]
      settings: DisplayOption=none
  Terminator1 : Terminator
  Terminator2 : Terminator
  Terminator3 : Terminator
  ypqr : Outport  Port=1
  wires:
  upqr/1 -> Demux/1
  Demux/1 -> Terminator3/1
  Demux/5 -> Terminator2/1
  Demux/3 -> Terminator1/1
  Demux/2 -> Fcn1/1, Fcn/1, Fcn2/1, Fcn4/1, Fcn5/1, Fcn3/1
  Demux/4 -> Mux/1
  Fcn/1 -> Mux/2
  Fcn1/1 -> Mux/3
  Fcn2/1 -> Mux/4
  Fcn3/1 -> Mux/5
  Fcn4/1 -> Mux/6
  Fcn5/1 -> Mux/7
  Matrix Gain/1 -> ypqr/1
  Mux/1 -> Matrix Gain/1

== system fdcwind/F4 Rearranged/FDC 6DoF/eqm/ODE/xyHdot ==
  note: yxyH=[xe dot; ye dot; H dot]
  note: uxyH=[x;Ftot;Mtot;yhlp]
  ybvel* : Inport  Port=1  PortWidth=-1  SampleTime=-1  DataType=auto
      settings: SignalType=auto
  uxYH : Inport  Port=2  PortWidth=-1  SampleTime=-1  DataType=auto
      settings: SignalType=auto
  0 : Subsystem
      settings: OpenFcn=fdchelp xyhdot
      mask Display: disp('XYHDOT\nM.O. Rauw, October 1997')
  H dot : Fcn  Expr=u[30]*u[26] - (u[31]*u[28]+u[32]*u[29])*u[27]
  Mux2 : Mux  Inputs=[29 3]
      settings: DisplayOption=none
  Mux3 : Mux  Inputs=2
      settings: DisplayOption=none
  Mux4 : Mux  Inputs=[29 2]
      settings: DisplayOption=none
  Mux5 : Mux  Inputs=3
      settings: DisplayOption=none
  tmp1 : Fcn  Expr=u[30]*u[27] + (u[31]*u[28]+u[32]*u[29])*u[26]
  tmp2 : Fcn  Expr=u[31]*u[29] - u[32]*u[28]
  xe dot : Fcn  Expr=u[30]*u[25] - u[31]*u[24]
  ye dot : Fcn  Expr=u[30]*u[24] + u[31]*u[25]
  yxyH : Outport  Port=1
  wires:
  tmp1/1 -> Mux3/1
  H dot/1 -> Mux5/3
  xe dot/1 -> Mux5/1
  tmp2/1 -> Mux3/2
  ye dot/1 -> Mux5/2
  Mux5/1 -> yxyH/1
  Mux4/1 -> ye dot/1, xe dot/1
  Mux2/1 -> H dot/1, tmp2/1, tmp1/1
  Mux3/1 -> Mux4/2
  ybvel*/1 -> Mux2/2
  uxYH/1 -> Mux4/1, Mux2/1

== system fdcwind/F4 Rearranged/FDC 6DoF/eqm/uvw/0 ==

== system fdcwind/F4 Rearranged/FDC 6DoF/out/accel/0 ==

== system fdcwind/F4 Rearranged/FDC 6DoF/out/fp/0 ==

== system fdcwind/F4 Rearranged/FDC 6DoF/out/uvwdot/0 ==

== system fdcwind/F4 Rearranged/FDC 6DoF/eqm/ODE/Eulerdot/0 ==

== system fdcwind/F4 Rearranged/FDC 6DoF/eqm/ODE/Vabdot/0 ==

== system fdcwind/F4 Rearranged/FDC 6DoF/eqm/ODE/pqrdot/0 ==

== system fdcwind/F4 Rearranged/FDC 6DoF/eqm/ODE/xyHdot/0 ==
